simulink model "rev2"  (R2018b)
settings: Solver=VariableStepAuto  StartTime=0.0  StopTime=60  RelTol=1e-3
PreLoadFcn:
  | % Import the data from Excel for a throttle-thrust lookup table
  | data = xlsread('ThrustVsThrottleDataset.xlsx');
  | % Row indices for lookup table
  | x = data(1:end,1)';
  | % Column indices for lookup table
  | y = transpose(data(1:end,3));
  | 
  | %remove duplicate points
  | breakpoints1=[];
  | breakpoints2=[];
  | count=0;
  | for i=2:length(x)
  |     previous=i-1;
  |     current=i;
  |     if x(current)~=x(previous)
  |         breakpoints1=[breakpoints1,x(previous)];
  |         breakpoints2=[breakpoints2,mean(y(previous:-1:previous-count))];
  |         count=0;
  |     else
  |         count=count+1;
  |     end
  | end
  | 
  | 
  | 
  | % Output values for lookup table
  | table_data = data(1:end,1:end);
libraries: simulink x1
settings Model: Creator=jchen  LastModifiedBy=jchen
settings SolverCC: ZeroCrossAlgorithm=Adaptive

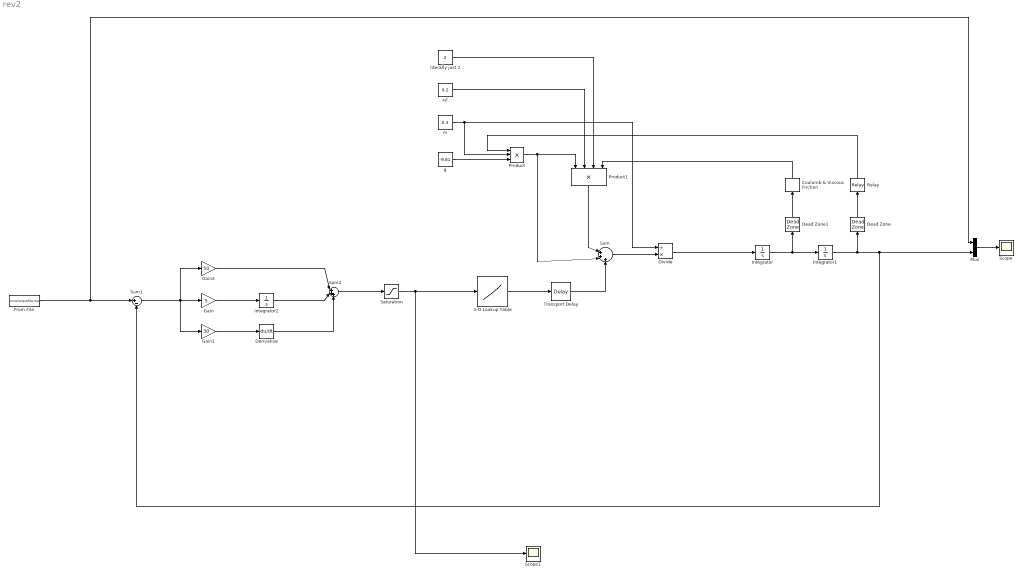
== system rev2 ==
  1-D Lookup Table : Lookup_n-D  NumberOfTableDimensions=1  BreakpointsForDimension1=breakpoints1  Table=breakpoints2  InternalRulePriority=Speed  RndMeth=Simplest  InputSameDT=on
  Coulomb & Viscous Friction : simulink/Discontinuities/Coulomb & Viscous Friction  offset=[0.13 0.13 0.13 0.13]  gain=0
      settings: SourceProductName=Simulink
  Dead Zone : DeadZone  LowerValue=-0.01  UpperValue=0.01  SaturateOnIntegerOverflow=on
  Dead Zone1 : DeadZone  LowerValue=-0.01  UpperValue=0.01  ZeroCross=off  SaturateOnIntegerOverflow=on
  Derivative : Derivative
  Divide : Product  Inputs=/*
  From File : FromFile  FileName=missionprofile.mat  SampleTime=0
  Gain : Gain  Gain=5
  Gain1 : Gain  Gain=30
  Gain2 : Gain  Gain=50
  Integrator : Integrator
  Integrator1 : Integrator
  Integrator2 : Integrator
  Mux : Mux  Inputs=2
  Product : Product  Inputs=3
  Product1 : Product  Inputs=4
  Relay : Relay  OnSwitchValue=0.001  OffSwitchValue=0
  Saturation : Saturate  UpperLimit=100  LowerLimit=0
  Scope : Scope
  Scope1 : Scope
  Sum : Sum  Inputs=|+++
  Sum1 : Sum  Inputs=|+-
  Sum2 : Sum  Inputs=|+++
  Transport Delay : TransportDelay  DelayTime=0.05
  g : Constant  Value=-9.81
  literally just 2 : Constant  Value=2
  m : Constant  Value=0.3
  "x/l " : Constant  Value=0.2
  wires:
  m/1 -> Product/2, Divide/1
  Product/1 -> Product1/1, Sum/2
  "x/l "/1 -> Product1/2
  literally just 2/1 -> Product1/3
  Product1/1 -> Sum/1
  Sum/1 -> Divide/2
  Divide/1 -> Integrator/1
  Integrator/1 -> Integrator1/1, Dead Zone1/1
  Coulomb & Viscous Friction/1 -> Product1/4
  Integrator1/1 -> Mux/2, Sum1/2, Dead Zone/1
  g/1 -> Product/3
  From File/1 -> Mux/1, Sum1/1
  Sum1/1 -> Gain1/1, Gain2/1, Gain/1
  Gain/1 -> Integrator2/1
  Gain1/1 -> Derivative/1
  Gain2/1 -> Sum2/1
  Integrator2/1 -> Sum2/2
  Derivative/1 -> Sum2/3
  Sum2/1 -> Saturation/1
  Saturation/1 -> 1-D Lookup Table/1, Scope1/1
  Mux/1 -> Scope/1
  Relay/1 -> Product/1
  Dead Zone/1 -> Relay/1
  Dead Zone1/1 -> Coulomb & Viscous Friction/1
  1-D Lookup Table/1 -> Transport Delay/1
  Transport Delay/1 -> Sum/3
